simulink model "teaching20260428"  (R2025b)
settings: Solver=VariableStepAuto  StartTime=0.0  StopTime=10.0  RelTol=1e-3
settings Model: Creator=itsyu  LastModifiedBy=itsyu

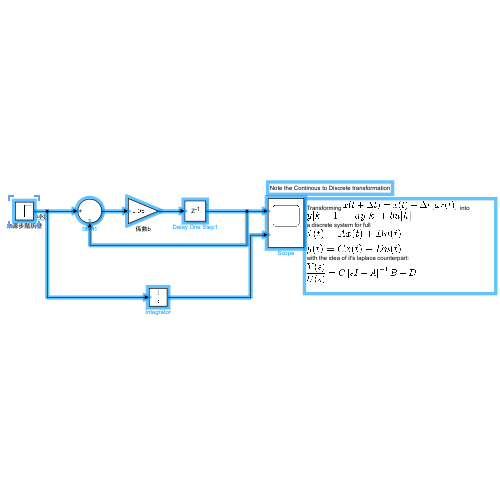
[thumbnail: Simulink's stored preview of the top-level diagram]
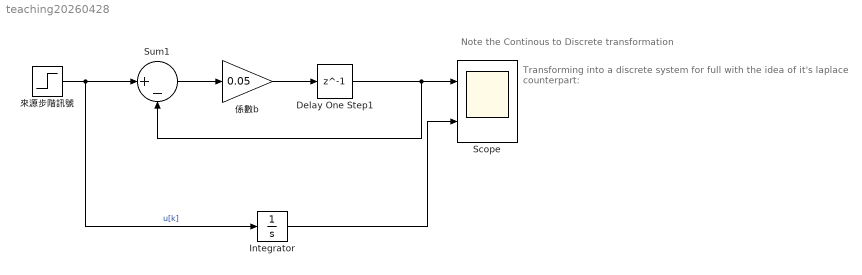
== system teaching20260428 ==
  note: Note the Continous to Discrete transformation
  note: Transforming into
      | a discrete system for full
      |
      | with the idea of it's laplace counterpart:
  Delay One Step1 : Delay  DelayLength=1
  Integrator : Integrator
  Scope : Scope  NumInputPorts=2
      settings: ActiveDisplayYMinimum=-0.62499999999999989  ActiveDisplayYMaximum=5.625
  Sum1 : Sum  Inputs=|+-
  來源步階訊號 : Step  Time=5  SampleTime=0
  係數b : Gain  Gain=0.05
  wires:
  係數b/1 -> Delay One Step1/1
  Delay One Step1/1 -> Sum1/2, Scope/1
  來源步階訊號/1 -> Integrator/1, Sum1/1  "u[k]"
  Sum1/1 -> 係數b/1
  Integrator/1 -> Scope/2
